simulink model "part2"  (R2023b)
settings: Solver=VariableStepAuto  StartTime=0.0  StopTime=500  RelTol=1e-3
values from neighbouring files (symbols this model uses):
  A = 1    [z_peng_exp_12_1.m]
  Cd = 0.5    [gemini.m]    (also in z_peng_exp_12_1.m)
  f = 0.015    [gemini.m]    (also in z_peng_exp_12_1.m)
  g = 9.81    [gemini.m]    (also in z_peng_exp_12_1.m)
  m = 1250    [gemini.m]    (also in z_peng_exp_12_1.m = 1000)
  m_eqv = m + I_w_total/r^2 + I_e*(G*R)^2/r^2    [gemini.m]
  ro = 1.225    [gemini.m]
libraries: simulink x2, simulink_extras x2, slpidlib x1, SignalEditorBlockLib x1
settings Model: Creator=yusufcagriogut  LastModifiedBy=yusufcagriogut

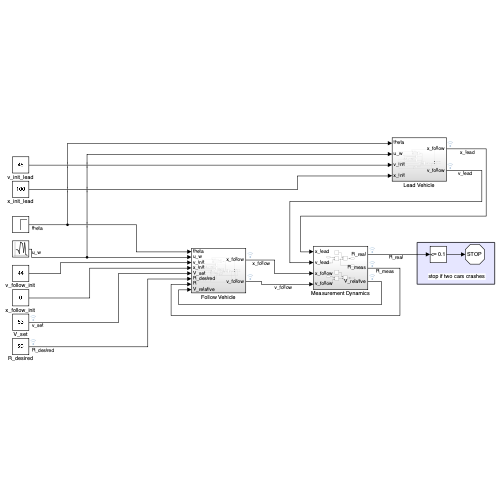
[thumbnail: Simulink's stored preview of the top-level diagram]
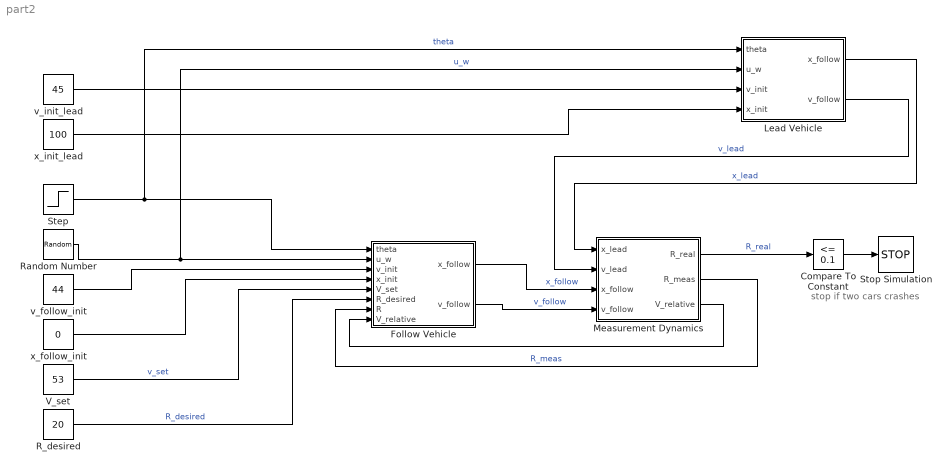
== system part2 ==
  note: stop if two cars crashes
  Compare To Constant : simulink/Logic and Bit Operations/Compare To Constant  relop=<=  const=0.1  OutDataTypeStr=boolean
  Follow Vehicle : Subsystem
  Lead Vehicle : Subsystem
  Measurement Dynamics : Subsystem
  R_desired : Constant  Value=20
  Random Number : RandomNumber  Variance=2  SampleTime=2
  Step : Step  Time=0  Before=3  After=3  SampleTime=0
  Stop Simulation : Stop
  V_set : Constant  Value=53
  v_follow_init : Constant  Value=44
  v_init_lead : Constant  Value=45
  x_follow_init : Constant  Value=0
  x_init_lead : Constant  Value=100
  wires:
  Lead Vehicle/2(v_follow) -> Measurement Dynamics/2(v_lead)  "v_lead"
  Lead Vehicle/1(x_follow) -> Measurement Dynamics/1(x_lead)  "x_lead"
  Measurement Dynamics/2(R_meas) -> Follow Vehicle/7(R)  "R_meas"
  Follow Vehicle/1(x_follow) -> Measurement Dynamics/3(x_follow)  "x_follow"
  Follow Vehicle/2(v_follow) -> Measurement Dynamics/4(v_follow)  "v_follow"
  Measurement Dynamics/3(V_relative) -> Follow Vehicle/8(V_relative)
  Step/1 -> Follow Vehicle/1(theta), Lead Vehicle/1(theta)  "theta"
  Random Number/1 -> Lead Vehicle/2(u_w), Follow Vehicle/2(u_w)  "u_w"
  v_init_lead/1 -> Lead Vehicle/3(v_init)
  x_init_lead/1 -> Lead Vehicle/4(x_init)
  v_follow_init/1 -> Follow Vehicle/3(v_init)
  x_follow_init/1 -> Follow Vehicle/4(x_init)
  Measurement Dynamics/1(R_real) -> Compare To Constant/1  "R_real"
  Compare To Constant/1 -> Stop Simulation/1
  V_set/1 -> Follow Vehicle/5(V_set)  "v_set"
  R_desired/1 -> Follow Vehicle/6(R_desired)  "R_desired"

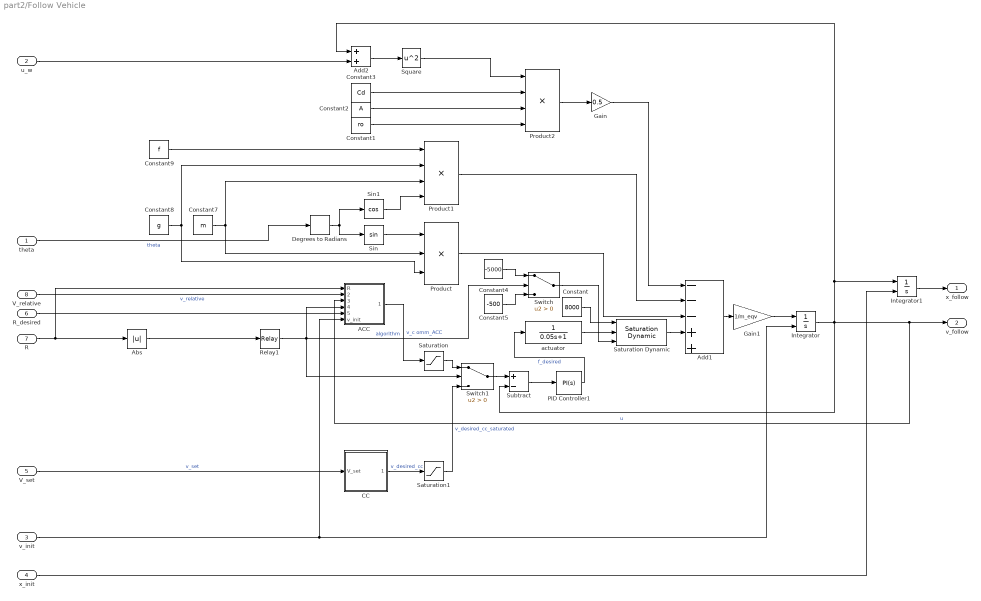
== system part2/Follow Vehicle ==
  theta : Inport
  u_w : Inport  Port=2
  v_init : Inport  Port=3
  x_init : Inport  Port=4
  V_set : Inport  Port=5
  R_desired : Inport  Port=6
  R : Inport  Port=7
  V_relative : Inport  Port=8
  ACC : Subsystem
  Abs : Abs  SaturateOnIntegerOverflow=off
  Add1 : Sum  Inputs=---++
  Add2 : Sum
  CC : Subsystem
  Constant : Constant  Value=8000
  Constant1 : Constant  Value=ro
  Constant2 : Constant  Value=A
  Constant3 : Constant  Value=Cd
  Constant4 : Constant  Value=-5000
  Constant5 : Constant  Value=-500
  Constant7 : Constant  Value=m
  Constant8 : Constant  Value=g
  Constant9 : Constant  Value=f
  Degrees to Radians : simulink_extras/Transformations/Degrees to Radians
  Gain : Gain  Gain=0.5
  Gain1 : Gain  Gain=1/m_eqv
  Integrator : Integrator  InitialConditionSource=external  InitialCondition=33
  Integrator1 : Integrator  InitialConditionSource=external
  PID Controller1 : slpidlib/PID Controller  Controller=PI  Form=Parallel  TimeDomain=Continuous-time  UseExternalTs=off  SampleTime=-1  IntegratorMethod=Forward Euler  FilterMethod=Forward Euler  ControllerParametersSource=internal  P=1900  I=50  UseKiTs=off  D=0  N=12.815158437423  UseFilter=on  TunerSelectOption=Transfer Function Based (PID Tuner App)  InitialConditionSource=internal  InitialConditionForIntegrator=0  InitialConditionForFilter=0  DifferentiatorICPrevScaledInput=0  ExternalReset=none  TrackingMode=off  Kt=1  LimitOutput=off  SatLimitsSource=internal  UpperSaturationLimit=inf  LowerSaturationLimit=-inf  LinearizeAsGain=on  AntiWindupMode=none  Kb=1  LimitIntegrator=off  UpperIntegratorSaturationLimit=inf  LowerIntegratorSaturationLimit=-inf  POutMin=[]  POutMax=[]  IOutMin=[]  IOutMax=[]  DOutMin=[]  DOutMax=[]  NOutMin=[]  NOutMax=[]  SumOutMin=[]  SumOutMax=[]  SaturationOutMin=[]  SaturationOutMax=[]  PParamMin=[]  PParamMax=[]  IParamMin=[]  IParamMax=[]  DParamMin=[]  DParamMax=[]  NParamMin=[]  NParamMax=[]  KbParamMin=[]  KbParamMax=[]  KtParamMin=[]  KtParamMax=[]  KbOutMin=[]  KbOutMax=[]  KtOutMin=[]  KtOutMax=[]  IntegratorOutMin=[]  IntegratorOutMax=[]  FilterOutMin=[]  FilterOutMax=[]  SumI1OutMin=[]  SumI1OutMax=[]  SumI2OutMin=[]  SumI2OutMax=[]  SumI3OutMin=[]  SumI3OutMax=[]  SumI4OutMin=[]  SumI4OutMax=[]  SumDOutMin=[]  SumDOutMax=[]  DifferentiatorOutMin=[]  DifferentiatorOutMax=[]  FilterDiffOutCoefMin=[]  FilterDiffOutCoefMax=[]  ReciprocalOutMin=[]  ReciprocalOutMax=[]  SumDenOutMin=[]  SumDenOutMax=[]  SumNumOutMin=[]  SumNumOutMax=[]  DivideOutMin=[]  DivideOutMax=[]  UdiffTsProdOutMin=[]  UdiffTsProdOutMax=[]  NTsProdOutMin=[]  NTsProdOutMax=[]  UintegralTsProdOutMin=[]  UintegralTsProdOutMax=[]  UngainTsProdOutMin=[]  UngainTsProdOutMax=[]  ClampingZeroOutDataTypeStr=Inherit: Inherit via back propagation  ClampingZeroOutMin=[]  ClampingZeroOutMax=[]  FilterDenConstantOutDataTypeStr=Inherit: Inherit via back propagation  FilterDenConstantOutMin=[]  FilterDenConstantOutMax=[]  PCopyOutDataTypeStr=Inherit: Inherit via back propagation  PCopyOutMin=[]  PCopyOutMax=[]  NCopyOutDataTypeStr=Inherit: Inherit via back propagation  NCopyOutMin=[]  NCopyOutMax=[]  IntegratorContinuousStateAttributes=''  IntegratorStateMustResolveToSignalObject=off  IntegratorRTWStateStorageClass=Auto  FilterContinuousStateAttributes=''  FilterStateMustResolveToSignalObject=off  FilterRTWStateStorageClass=Auto  ParallelPVariant=InternalParameters  IdealPVariant=Disabled  IVariant=InternalParameters  DVariant=Disabled  IntegratorVariant=Continuous  SatVariant=Disabled  AWVariant=Passthrough  PCopyVariant=Disabled  TRVariant=Disabled  FdbkBlocksVariant=Forward  IdealPFdbkVariant=Disabled  SatFdbkVariant=Disabled  DerivativeFilterVariant=Disabled  NVariant=Disabled  NCopyVariant=Disabled_SignalSpec  FilterICVariant=Disabled  IntegratorICVariant=InternalICs  ExternalResetVariant=Disabled  TRSumVariant=Passthrough  SumFdbkVariant=Disabled  SumVariant=Sum_PI  TsampFilterVariant=InternalTs  TsampNgainVariant=Passthrough  TsampIntegralVariant=Disabled_SignalSpec  ExternalSaturationOutDataTypeStr=Inherit: Same as second input
  Product : Product  Inputs=3
  Product1 : Product  Inputs=4
  Product2 : Product  Inputs=4
  Relay1 : Relay  OnSwitchValue=35  OffSwitchValue=20  OnOutputValue=0  OffOutputValue=1
  Saturation : Saturate  UpperLimit=50  LowerLimit=0
  Saturation Dynamic : simulink/Discontinuities/Saturation Dynamic  OutMin=[]  OutMax=[]  OutDataTypeStr=Inherit: Same as second input  OutDataType=fixdt(1, 16)  OutScaling=2^-10  DoSatur=off
  Saturation1 : Saturate  UpperLimit=50  LowerLimit=0
  Sin : Trigonometry
  Sin1 : Trigonometry  Operator=cos
  Square : Math  Operator=square
  Subtract : Sum  Inputs=+-
  Switch : Switch  Criteria=u2 > Threshold  SaturateOnIntegerOverflow=off  InputSameDT=off
  Switch1 : Switch  Criteria=u2 > Threshold  SaturateOnIntegerOverflow=off  InputSameDT=off
  actuator : TransferFcn  Denominator=[0.05 1]
  x_follow : Outport
  v_follow : Outport  Port=2
  wires:
  Integrator1/1 -> x_follow/1
  R/1 -> ACC/1(R), Abs/1
  Abs/1 -> Relay1/1
  Gain1/1 -> Integrator/1
  Add1/1 -> Gain1/1
  actuator/1 -> Saturation Dynamic/2
  Product2/1 -> Gain/1
  Add2/1 -> Square/1
  Constant1/1 -> Product2/4
  Constant2/1 -> Product2/3
  Constant3/1 -> Product2/2
  u_w/1 -> Add2/2
  Square/1 -> Product2/1
  Integrator/1 -> Subtract/2, ACC/3(V_follow), v_follow/1, Integrator1/1, Add2/1  "u"
  Gain/1 -> Add1/1
  theta/1 -> Degrees to Radians/1  "theta"
  Sin/1 -> Product/1
  Product/1 -> Add1/3
  Constant8/1 -> Product/3, Product1/2
  Sin1/1 -> Product1/4
  Constant7/1 -> Product/2, Product1/3
  Product1/1 -> Add1/2
  Constant9/1 -> Product1/1
  Degrees to Radians/1 -> Sin/1, Sin1/1
  v_init/1 -> ACC/6(v_init), Integrator/2
  x_init/1 -> Integrator1/2
  V_relative/1 -> ACC/2(V_relative)  "v_relative"
  V_set/1 -> CC/1(V_set)  "v_set"
  Saturation/1 -> Switch1/1
  ACC/1(v_desired) -> Saturation/1  "v_c omm_ACC"
  Switch1/1 -> Subtract/1
  CC/1(V_desired) -> Saturation1/1  "v_desired_cc"
  Saturation1/1 -> Switch1/3  "v_desired_cc_saturated"
  R_desired/1 -> ACC/5(R_desired)
  Constant4/1 -> Switch/1
  Constant5/1 -> Switch/3
  Saturation Dynamic/1 -> Add1/4
  Constant/1 -> Saturation Dynamic/1
  Switch/1 -> Saturation Dynamic/3
  PID Controller1/1 -> actuator/1  "f_desired"
  Subtract/1 -> PID Controller1/1
  Relay1/1 -> Switch/2, ACC/4(active), Switch1/2  "algorithm"

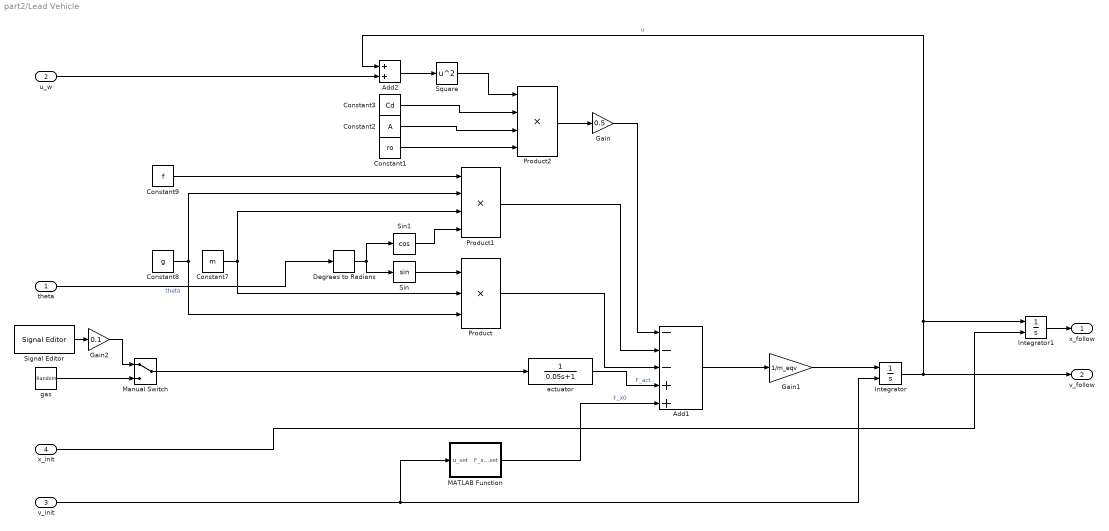
== system part2/Lead Vehicle ==
  theta : Inport
  u_w : Inport  Port=2
  v_init : Inport  Port=3
  x_init : Inport  Port=4
  Add1 : Sum  Inputs=---++
  Add2 : Sum
  Constant1 : Constant  Value=ro
  Constant2 : Constant  Value=A
  Constant3 : Constant  Value=Cd
  Constant7 : Constant  Value=m
  Constant8 : Constant  Value=g
  Constant9 : Constant  Value=f
  Degrees to Radians : simulink_extras/Transformations/Degrees to Radians
  Gain : Gain  Gain=0.5
  Gain1 : Gain  Gain=1/m_eqv
  Gain2 : Gain  Gain=0.1
  Integrator : Integrator  InitialConditionSource=external  InitialCondition=33
  Integrator1 : Integrator  InitialConditionSource=external
  MATLAB Function : MATLAB Function  TreatAsAtomicUnit=on
  Manual Switch : ManualSwitch
  Product : Product  Inputs=3
  Product1 : Product  Inputs=4
  Product2 : Product  Inputs=4
  Signal Editor : SignalEditorBlockLib/Signal Editor  FileName=leadcar_force.mat  ActiveScenario=Scenario  ActiveSignal=Signal 1  IsBus=off  OutputBusObjectStr=Bus: BusObject  SampleTime=0  Interpolate=off  ZeroCross=off  OutputAfterFinalValue=Setting to zero  Unit=inherit  PreserveSignalName=on  ApplySigPropsToAllScenarios=on  ApplySigPropsToAllSignals=off
  Sin : Trigonometry
  Sin1 : Trigonometry  Operator=cos
  Square : Math  Operator=square
  actuator : TransferFcn  Denominator=[0.05 1]
  gas : RandomNumber  Variance=5000  SampleTime=2
  x_follow : Outport
  v_follow : Outport  Port=2
  wires:
  Integrator1/1 -> x_follow/1
  Gain1/1 -> Integrator/1
  Add1/1 -> Gain1/1
  v_init/1 -> MATLAB Function/1(u_set), Integrator/2
  actuator/1 -> Add1/4  "F_act"
  Product2/1 -> Gain/1
  Add2/1 -> Square/1
  Constant1/1 -> Product2/4
  Constant2/1 -> Product2/3
  Constant3/1 -> Product2/2
  u_w/1 -> Add2/2
  Square/1 -> Product2/1
  Integrator/1 -> Integrator1/1, Add2/1, v_follow/1  "u"
  Gain/1 -> Add1/1
  theta/1 -> Degrees to Radians/1  "theta"
  Sin/1 -> Product/1
  Product/1 -> Add1/3
  Constant8/1 -> Product/3, Product1/2
  Sin1/1 -> Product1/4
  Constant7/1 -> Product/2, Product1/3
  Product1/1 -> Add1/2
  Constant9/1 -> Product1/1
  Degrees to Radians/1 -> Sin/1, Sin1/1
  x_init/1 -> Integrator1/2
  MATLAB Function/1(F_x0_set) -> Add1/5  "F_x0"
  Manual Switch/1 -> actuator/1
  gas/1 -> Manual Switch/2
  Signal Editor/1 -> Gain2/1
  Gain2/1 -> Manual Switch/1

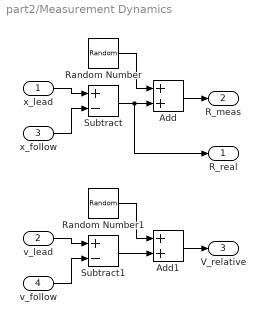
== system part2/Measurement Dynamics ==
  x_lead : Inport
  v_lead : Inport  Port=2
  x_follow : Inport  Port=3
  v_follow : Inport  Port=4
  Add : Sum
  Add1 : Sum
  Random Number : RandomNumber  Variance=0.2  SampleTime=0.1
  Random Number1 : RandomNumber  Variance=0.1  SampleTime=0.1
  Subtract : Sum  Inputs=+-
  Subtract1 : Sum  Inputs=+-
  R_real : Outport
  R_meas : Outport  Port=2
  V_relative : Outport  Port=3
  wires:
  Add/1 -> R_meas/1
  x_lead/1 -> Subtract/1
  x_follow/1 -> Subtract/2
  Subtract/1 -> R_real/1, Add/2
  Random Number/1 -> Add/1
  Add1/1 -> V_relative/1
  Subtract1/1 -> Add1/2
  Random Number1/1 -> Add1/1
  v_follow/1 -> Subtract1/2
  v_lead/1 -> Subtract1/1

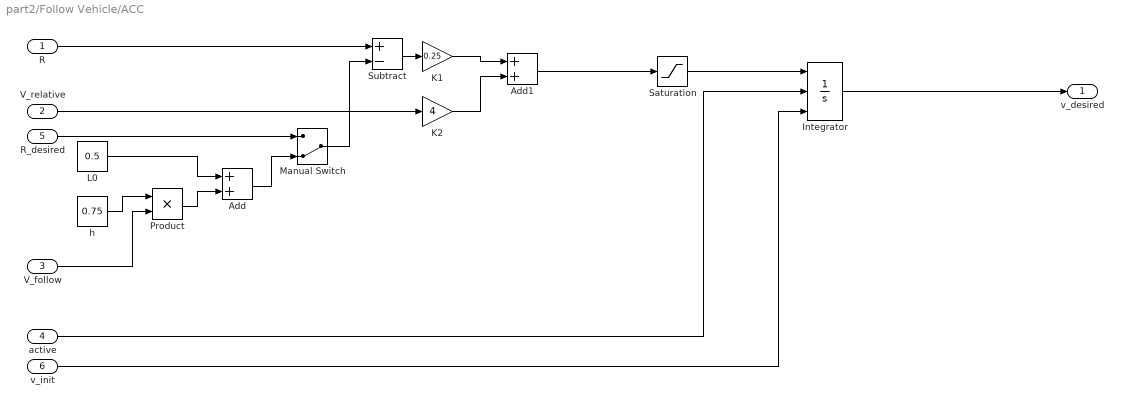
== system part2/Follow Vehicle/ACC ==
  R : Inport
  V_relative : Inport  Port=2
  V_follow : Inport  Port=3
  active : Inport  Port=4
  R_desired : Inport  Port=5
  v_init : Inport  Port=6
  Add : Sum
  Add1 : Sum
  Integrator : Integrator  ExternalReset=rising  InitialConditionSource=external  LimitOutput=on  UpperSaturationLimit=50  LowerSaturationLimit=0
  K1 : Gain  Gain=0.25
  K2 : Gain  Gain=4
  L0 : Constant  Value=0.5
  Manual Switch : ManualSwitch  CurrentSetting=0
  Product : Product
  Saturation : Saturate  UpperLimit=2.5  LowerLimit=-1
  Subtract : Sum  Inputs=+-
  h : Constant  Value=0.75
  v_desired : Outport
  wires:
  R/1 -> Subtract/1
  h/1 -> Product/1
  V_follow/1 -> Product/2
  L0/1 -> Add/1
  Product/1 -> Add/2
  Subtract/1 -> K1/1
  V_relative/1 -> K2/1
  K1/1 -> Add1/1
  Add1/1 -> Saturation/1
  active/1 -> Integrator/2
  R_desired/1 -> Manual Switch/1
  K2/1 -> Add1/2
  v_init/1 -> Integrator/3
  Add/1 -> Manual Switch/2
  Manual Switch/1 -> Subtract/2
  Saturation/1 -> Integrator/1
  Integrator/1 -> v_desired/1

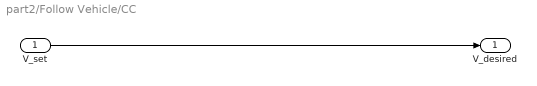
== system part2/Follow Vehicle/CC ==
  V_set : Inport
  V_desired : Outport
  wires:
  V_set/1 -> V_desired/1

== matlab function part2/Lead Vehicle/MATLAB Function ==
  data: u_set input; F_x0_set output
function F_x0_set = fcn(u_set)
m = 1250;
ro = 1.225;
A = 1.2;
Cd = 0.5;
f = 0.015;
R = 3;
I_e = 0.15;
r = 0.3;
I_w = 1.0;
u_0 = 40;
u_w = 2;
g = 9.81;
theta_0 = 0;
F_x0_set = m*g*sin(theta_0) + f*m*g*cos(theta_0) + ...
    0.5*ro*A*Cd*(u_set+u_w)^2;
end
